simulink model "TD3"  (Simulink 8.3)
settings: Solver=ode45  StartTime=0.0  StopTime=600  RelTol=1e-3
values from neighbouring files (symbols this model uses):
  a1 = 0    [TD3init.m]
  a2 = 0    [TD3init.m]
  b1 = 1    [TD3init.m]
  b2 = 1    [TD3init.m]
  c1 = 0    [TD3init.m]
  c2 = 0    [TD3init.m]
  d1 = 1    [TD3init.m]
  d2 = 1    [TD3init.m]
  k = 1.2    [TD3init.m]
  kc = 4.2    [TD3init.m]
  T1 = 155    [TD3init.m]
  T2 = 2    [TD3init.m]
  Td = 51    [TD3init.m]
  Te = 60    [TD3init.m]
  Tfi = 37    [TD3init.m]
  Ti = 273    [TD3init.m]
settings Model: Creator=bassot  LastModifiedBy=bassot
settings OptimizationCC: ExpressionDepthLimit=2147483647  InitFltsAndDblsToZero=on
settings DebuggingCC: SaveWithParameterizedLinksMsg=none  SignalResolutionControl=TryResolveAllWithWarning  MultiTaskDSMMsg=warning  MultiTaskCondExecSysMsg=none  FcnCallInpInsideContextMsg=UseLocalSettings
settings RTWCC: IncludeERTFirstTime=on
settings GRTTargetCC: TargetFcnLib=ansi_tfl_tmw.mat

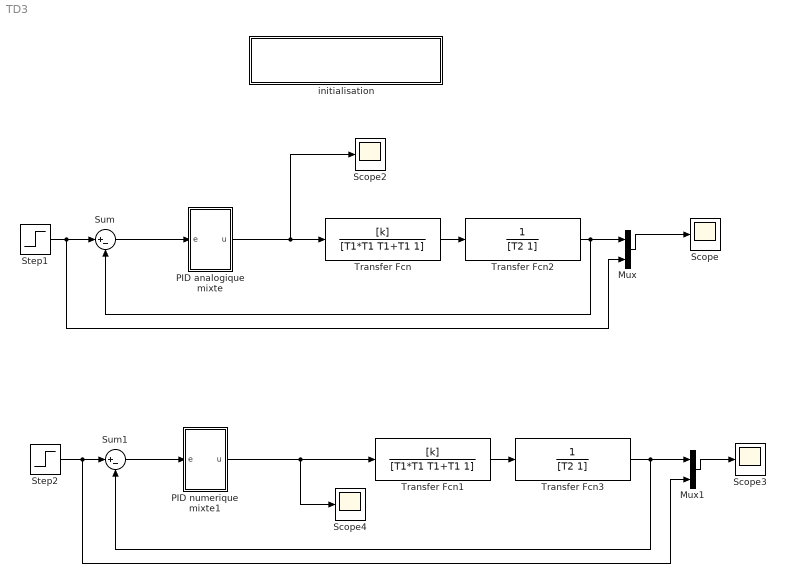
== system TD3 ==
  " PID analogique mixte" : Subsystem
  " PID numerique mixte1" : Subsystem
  Mux : Mux  Inputs=2
  Mux1 : Mux  Inputs=2
  Scope{,2..4} (4 alike) : Scope
      Scope settings: TimeRange=2000
      Scope2 settings: TimeRange=2000  SaveName=ScopeData2
      Scope3 settings: TimeRange=2000  SaveName=ScopeData3
      Scope4 settings: TimeRange=2000  SaveName=ScopeData4
  Step1 : Step  Time=0  After=20  SampleTime=0
  Step2 : Step  Time=0  After=20  SampleTime=0
  Sum : Sum  Inputs=|+-
  Sum1 : Sum  Inputs=|+-
  Transfer Fcn : TransferFcn  Numerator=[k]  Denominator=[T1*T1 T1+T1 1]
  Transfer Fcn1 : TransferFcn  Numerator=[k]  Denominator=[T1*T1 T1+T1 1]
  Transfer Fcn2 : TransferFcn  Denominator=[T2 1]
  Transfer Fcn3 : TransferFcn  Denominator=[T2 1]
  initialisation : Subsystem  TreatAsAtomicUnit=on
      settings: OpenFcn=TD3init
      mask Display: disp('double clic pour  \nexecuter TD3init')
  wires:
  Step1/1 -> Mux/2, Sum/1
  Mux/1 -> Scope/1
  Sum/1 -> " PID analogique mixte"/1(e)
  " PID analogique mixte"/1(u) -> Transfer Fcn/1, Scope2/1
  Mux1/1 -> Scope3/1
  Sum1/1 -> " PID numerique mixte1"/1(e)
  " PID numerique mixte1"/1(u) -> Transfer Fcn1/1, Scope4/1
  Transfer Fcn/1 -> Transfer Fcn2/1
  Transfer Fcn2/1 -> Mux/1, Sum/2
  Transfer Fcn1/1 -> Transfer Fcn3/1
  Transfer Fcn3/1 -> Mux1/1, Sum1/2
  Step2/1 -> Mux1/2, Sum1/1

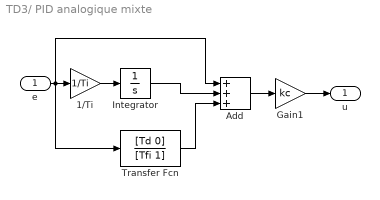
== system TD3/ PID analogique mixte ==
  e : Inport
  1/Ti : Gain  Gain=1/Ti
  Add : Sum  Inputs=+++
  Gain1 : Gain  Gain=kc
  Integrator : Integrator
  Transfer Fcn : TransferFcn  Numerator=[Td 0]  Denominator=[Tfi 1]
  u : Outport
  wires:
  Transfer Fcn/1 -> Add/3
  Integrator/1 -> Add/2
  1/Ti/1 -> Integrator/1
  e/1 -> Add/1, Transfer Fcn/1, 1/Ti/1
  Add/1 -> Gain1/1
  Gain1/1 -> u/1

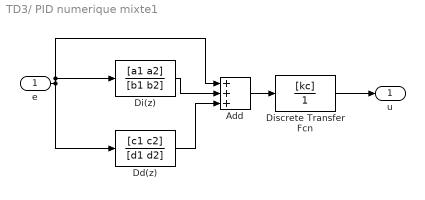
== system TD3/ PID numerique mixte1 ==
  e : Inport
  Add : Sum  Inputs=+++
  Dd(z) : DiscreteTransferFcn  Numerator=[c1 c2]  Denominator=[d1 d2]  SampleTime=Te
  Di(z) : DiscreteTransferFcn  Numerator=[a1 a2]  Denominator=[b1 b2]  SampleTime=Te
  Discrete Transfer Fcn : DiscreteTransferFcn  Numerator=[kc]  Denominator=[1]  SampleTime=Te
  u : Outport
  wires:
  Dd(z)/1 -> Add/3
  Di(z)/1 -> Add/2
  e/1 -> Add/1, Di(z)/1, Dd(z)/1
  Add/1 -> Discrete Transfer Fcn/1
  Discrete Transfer Fcn/1 -> u/1

== system TD3/initialisation ==
